simulink model "my_buck_nn_5_10"  (R2021a)
settings: Solver=ode8  StartTime=0.0  StopTime=T  RelTol=1e-3  EnableMultiTasking=on
undefined symbols (not defined in the file): a00c, a00o, a01c, a01o, a10c, a10o, a11c, a11o, b0c, b0o, b1c, b1o, i0, T_sw, v0
libraries: neural x57, simulink x1
(part 2 of 2)

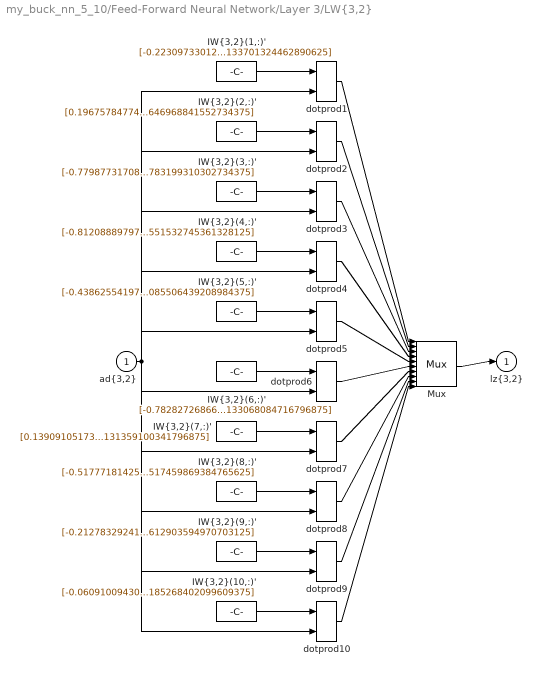
== system my_buck_nn_5_10/Feed-Forward Neural Network/Layer 3/LW{3,2} ==
  "ad{3,2}" : Inport  PortDimensions=10
      mask Display: e = 0.06;c1 = [120 230 180]/255;c2 = ([120 230 180]+0)/(256+128);c3 = ([120 230 180]+128)/(256+128);patch([0 1 1 0],[0 0 1 1],c1);patch([0 1 1 1-e 1-e 0+e],[0 0 1 1-e 0+e 0+e],c2);patch([0 0 1 1-e 0+e 0+e],[0 1 1 1-e 1-e 0+e],c3);plot([0 1 1 0 0],[0 0 1 1 0]);
  "IW{3,2}(1,:)'" : Constant  Value=[-0.2230973301246004236730868797167204320430755615234375;-0.7932748282150023921843740026815794408321380615234375;0.79085097892476452496879346654168330132961273193359375;-0.70189923383787033994707371675758622586727142333984375;-0.989793512776859785162741900421679019927978515625;-0.25570181827175486599657006081542931497097015380859375;-0.4845417555697097977684961733757518231868743896484375;-0.03901169535660164999768539928481914103031158447265625;-0.1497645933363858095077603138634003698825836181640625;0.5126260157213560209044089788221754133701324462890625]
      mask Display: e = 0.06;c1 = [120 150 230]/255;c2 = ([120 150 230]+0)/383;c3 = ([120 150 230]+128)/383;patch([0 1 1 0],[0 0 1 1],c1);patch([0 1 1 1-e 1-e 0+e],[0 0 1 1-e 0+e 0+e],c2);patch([0 0 1 1-e 0+e 0+e],[0 1 1 1-e 1-e 0+e],c3);plot([0 1 1 0 0],[0 0 1 1 0]);disp('weights');
  "IW{3,2}(10,:)'" : Constant  Value=[-0.0609100943023948016019630813389085233211517333984375;-0.80372367245294196180793733219616115093231201171875;0.27081599181474358406518376796157099306583404541015625;0.265189392929031431123121365089900791645050048828125;-0.7240301944141958045975115965120494365692138671875;-0.57188810753222940608253566097118891775608062744140625;0.55258359868805495551669082487933337688446044921875;-0.40945653303743967388328428569366224110126495361328125;-0.7914296649209917600131802828400395810604095458984375;-0.33082945599161239780272580901510082185268402099609375]
      mask Display: e = 0.06;c1 = [120 150 230]/255;c2 = ([120 150 230]+0)/383;c3 = ([120 150 230]+128)/383;patch([0 1 1 0],[0 0 1 1],c1);patch([0 1 1 1-e 1-e 0+e],[0 0 1 1-e 0+e 0+e],c2);patch([0 0 1 1-e 0+e 0+e],[0 1 1 1-e 1-e 0+e],c3);plot([0 1 1 0 0],[0 0 1 1 0]);disp('weights');
  "IW{3,2}(2,:)'" : Constant  Value=[0.196757847742274893931835322291590273380279541015625;0.6454480727285536456605541388853453099727630615234375;0.99750915171941356707208115039975382387638092041015625;0.827041936661400800545607125968672335147857666015625;0.0417420581953746872017063651583157479763031005859375;1.0293967746717260780542346765287220478057861328125;0.00641324259274966834709630347788333892822265625;-0.09573473684369075697997431007024715654551982879638671875;-0.2787173553106720991223710370832122862339019775390625;-0.260939600114958147880628303028061054646968841552734375]
      mask Display: e = 0.06;c1 = [120 150 230]/255;c2 = ([120 150 230]+0)/383;c3 = ([120 150 230]+128)/383;patch([0 1 1 0],[0 0 1 1],c1);patch([0 1 1 1-e 1-e 0+e],[0 0 1 1-e 0+e 0+e],c2);patch([0 0 1 1-e 0+e 0+e],[0 1 1 1-e 1-e 0+e],c3);plot([0 1 1 0 0],[0 0 1 1 0]);disp('weights');
  "IW{3,2}(3,:)'" : Constant  Value=[-0.779877317085582166811263959971256554126739501953125;-0.310071870090603274316976012414670549333095550537109375;0.72432386795238923316020418496918864548206329345703125;0.419290922552696176950348672107793390750885009765625;-0.56736289194307421013263592612929642200469970703125;-0.3526319020860426700636480745743028819561004638671875;0.3565431330236761287011404419899918138980865478515625;1.246137269856822715752286967472173273563385009765625;-0.8664588759141953477893594026681967079639434814453125;0.1539704729454270670796489639542414806783199310302734375]
      mask Display: e = 0.06;c1 = [120 150 230]/255;c2 = ([120 150 230]+0)/383;c3 = ([120 150 230]+128)/383;patch([0 1 1 0],[0 0 1 1],c1);patch([0 1 1 1-e 1-e 0+e],[0 0 1 1-e 0+e 0+e],c2);patch([0 0 1 1-e 0+e 0+e],[0 1 1 1-e 1-e 0+e],c3);plot([0 1 1 0 0],[0 0 1 1 0]);disp('weights');
  "IW{3,2}(4,:)'" : Constant  Value=[-0.8120888979725917611318664057762362062931060791015625;0.6989923138619509312974287240649573504924774169921875;-0.8092821167810611004966858672560192644596099853515625;0.9321006564887095446891862593474797904491424560546875;-0.47196353282645731042066472582519054412841796875;-0.7802084968839901879533726969384588301181793212890625;0.5970384044771872567025639000348746776580810546875;0.695697603264001873668576081399805843830108642578125;-0.657985029570661961173527743085287511348724365234375;-0.92353117770848058842858563366462476551532745361328125]
      mask Display: e = 0.06;c1 = [120 150 230]/255;c2 = ([120 150 230]+0)/383;c3 = ([120 150 230]+128)/383;patch([0 1 1 0],[0 0 1 1],c1);patch([0 1 1 1-e 1-e 0+e],[0 0 1 1-e 0+e 0+e],c2);patch([0 0 1 1-e 0+e 0+e],[0 1 1 1-e 1-e 0+e],c3);plot([0 1 1 0 0],[0 0 1 1 0]);disp('weights');
  "IW{3,2}(5,:)'" : Constant  Value=[-0.438625541976773281049872821313329041004180908203125;-0.83434166362172679232145355854299850761890411376953125;-0.10138351170699401448960230709417373873293399810791015625;-0.7312618806762001266719153136364184319972991943359375;-0.290691564768943866425843225442804396152496337890625;-0.03730485749667165895626652627470321021974086761474609375;0.502479013885176239995189462206326425075531005859375;0.445592640810527129691109848863561637699604034423828125;0.53963122023129361792825875454582273960113525390625;-0.75669893589882464279838814036338590085506439208984375]
      mask Display: e = 0.06;c1 = [120 150 230]/255;c2 = ([120 150 230]+0)/383;c3 = ([120 150 230]+128)/383;patch([0 1 1 0],[0 0 1 1],c1);patch([0 1 1 1-e 1-e 0+e],[0 0 1 1-e 0+e 0+e],c2);patch([0 0 1 1-e 0+e 0+e],[0 1 1 1-e 1-e 0+e],c3);plot([0 1 1 0 0],[0 0 1 1 0]);disp('weights');
  "IW{3,2}(6,:)'" : Constant  Value=[-0.7828272686657609114035949460230767726898193359375;-0.8950889462309967736786120440228842198848724365234375;0.96021626961651695975064058075076900422573089599609375;-0.4361700008671605122145820132573135197162628173828125;-0.72811329607470209879238609573803842067718505859375;0.78059976706595379791764344190596602857112884521484375;-0.0663312268493079226772124457056634128093719482421875;-0.4842613379382820770757689388119615614414215087890625;0.914253204482205372727321446291171014308929443359375;-0.90156556177200986024189433010178618133068084716796875]
      mask Display: e = 0.06;c1 = [120 150 230]/255;c2 = ([120 150 230]+0)/383;c3 = ([120 150 230]+128)/383;patch([0 1 1 0],[0 0 1 1],c1);patch([0 1 1 1-e 1-e 0+e],[0 0 1 1-e 0+e 0+e],c2);patch([0 0 1 1-e 0+e 0+e],[0 1 1 1-e 1-e 0+e],c3);plot([0 1 1 0 0],[0 0 1 1 0]);disp('weights');
  "IW{3,2}(7,:)'" : Constant  Value=[0.13909105173843716585224683512933552265167236328125;0.75522199756791630331775877493782900273799896240234375;0.9269594132792653429220308680669404566287994384765625;-0.925064417004890504614422752638347446918487548828125;0.9889470498369294926277461854624561965465545654296875;0.99295289620838256272605804042541421949863433837890625;-0.381661240820658775874107959680259227752685546875;-0.50378735118134054804528432214283384382724761962890625;0.471059893245600047606558291590772569179534912109375;-0.73205460720426163145901909956592135131359100341796875]
      mask Display: e = 0.06;c1 = [120 150 230]/255;c2 = ([120 150 230]+0)/383;c3 = ([120 150 230]+128)/383;patch([0 1 1 0],[0 0 1 1],c1);patch([0 1 1 1-e 1-e 0+e],[0 0 1 1-e 0+e 0+e],c2);patch([0 0 1 1-e 0+e 0+e],[0 1 1 1-e 1-e 0+e],c3);plot([0 1 1 0 0],[0 0 1 1 0]);disp('weights');
  "IW{3,2}(8,:)'" : Constant  Value=[-0.5177718142514573518297993359738029539585113525390625;0.58233364417824284853253402616246603429317474365234375;-0.82418594893296648340452748016105033457279205322265625;-0.1877319934952508539982574120585923083126544952392578125;-0.1058780985460454626689852375420741736888885498046875;-0.450030200081221576358103675374877639114856719970703125;0.2461491554452306385059046078822575509548187255859375;0.8445581490884281894437890514382161200046539306640625;-0.06654864536490290305437156348489224910736083984375;0.5417979307102049890687567312852479517459869384765625]
      mask Display: e = 0.06;c1 = [120 150 230]/255;c2 = ([120 150 230]+0)/383;c3 = ([120 150 230]+128)/383;patch([0 1 1 0],[0 0 1 1],c1);patch([0 1 1 1-e 1-e 0+e],[0 0 1 1-e 0+e 0+e],c2);patch([0 0 1 1-e 0+e 0+e],[0 1 1 1-e 1-e 0+e],c3);plot([0 1 1 0 0],[0 0 1 1 0]);disp('weights');
  "IW{3,2}(9,:)'" : Constant  Value=[-0.2127832924122099456099022063426673412322998046875;0.0299459590999605375361003467560294666327536106109619140625;-0.351824095765843558591967621396179310977458953857421875;-0.9245459727240372682643965163151733577251434326171875;0.62369822352246284680177268455736339092254638671875;0.90248600905930087545669948667637072503566741943359375;-0.5037594788739097051433191154501400887966156005859375;0.385035381831421774645463074193685315549373626708984375;-0.4523169523443575368304436778998933732509613037109375;0.333631398082735952659305667111766524612903594970703125]
      mask Display: e = 0.06;c1 = [120 150 230]/255;c2 = ([120 150 230]+0)/383;c3 = ([120 150 230]+128)/383;patch([0 1 1 0],[0 0 1 1],c1);patch([0 1 1 1-e 1-e 0+e],[0 0 1 1-e 0+e 0+e],c2);patch([0 0 1 1-e 0+e 0+e],[0 1 1 1-e 1-e 0+e],c3);plot([0 1 1 0 0],[0 0 1 1 0]);disp('weights');
  Mux : Mux  Inputs=10
      mask Display: e = 0.06;c1 = [120 150 230]/255;c2 = ([120 150 230]+0)/383;c3 = ([120 150 230]+128)/383;patch([0 1 1 0],[0 0 1 1],c1);patch([0 1 1 1-e 1-e 0+e],[0 0 1 1-e 0+e 0+e],c2);patch([0 0 1 1-e 0+e 0+e],[0 1 1 1-e 1-e 0+e],c3);plot([0 1 1 0 0],[0 0 1 1 0]);disp('Mux');
  dotprod{1..10} (10 alike) : neural/Weight Functions/dotprod
  "lz{3,2}" : Outport
      mask Display: e = 0.06;c1 = [120 230 180]/255;c2 = ([120 230 180]+0)/(256+128);c3 = ([120 230 180]+128)/(256+128);patch([0 1 1 0],[0 0 1 1],c1);patch([0 1 1 1-e 1-e 0+e],[0 0 1 1-e 0+e 0+e],c2);patch([0 0 1 1-e 0+e 0+e],[0 1 1 1-e 1-e 0+e],c3);plot([0 1 1 0 0],[0 0 1 1 0]);
  wires:
  "IW{3,2}(1,:)'"/1 -> dotprod1/1
  "ad{3,2}"/1 -> dotprod1/2, dotprod2/2, dotprod3/2, dotprod4/2, dotprod5/2, dotprod6/2, dotprod7/2, dotprod8/2, dotprod9/2, dotprod10/2
  dotprod1/1 -> Mux/1
  "IW{3,2}(2,:)'"/1 -> dotprod2/1
  dotprod2/1 -> Mux/2
  "IW{3,2}(3,:)'"/1 -> dotprod3/1
  dotprod3/1 -> Mux/3
  "IW{3,2}(4,:)'"/1 -> dotprod4/1
  dotprod4/1 -> Mux/4
  "IW{3,2}(5,:)'"/1 -> dotprod5/1
  dotprod5/1 -> Mux/5
  "IW{3,2}(6,:)'"/1 -> dotprod6/1
  dotprod6/1 -> Mux/6
  "IW{3,2}(7,:)'"/1 -> dotprod7/1
  dotprod7/1 -> Mux/7
  "IW{3,2}(8,:)'"/1 -> dotprod8/1
  dotprod8/1 -> Mux/8
  "IW{3,2}(9,:)'"/1 -> dotprod9/1
  dotprod9/1 -> Mux/9
  "IW{3,2}(10,:)'"/1 -> dotprod10/1
  dotprod10/1 -> Mux/10
  Mux/1 -> "lz{3,2}"/1

== system my_buck_nn_5_10/Feed-Forward Neural Network/Layer 4/Delays 1 ==
  "p{4}" : Inport  PortDimensions=10
      mask Display: e = 0.06;c1 = [120 230 180]/255;c2 = ([120 230 180]+0)/(256+128);c3 = ([120 230 180]+128)/(256+128);patch([0 1 1 0],[0 0 1 1],c1);patch([0 1 1 1-e 1-e 0+e],[0 0 1 1-e 0+e 0+e],c2);patch([0 0 1 1-e 0+e 0+e],[0 1 1 1-e 1-e 0+e],c3);plot([0 1 1 0 0],[0 0 1 1 0]);
  mux : Mux  Inputs=1
      mask Display: e = 0.06;c1 = [120 150 230]/255;c2 = ([120 150 230]+0)/383;c3 = ([120 150 230]+128)/383;patch([0 1 1 0],[0 0 1 1],c1);patch([0 1 1 1-e 1-e 0+e],[0 0 1 1-e 0+e 0+e],c2);patch([0 0 1 1-e 0+e 0+e],[0 1 1 1-e 1-e 0+e],c3);plot([0 1 1 0 0],[0 0 1 1 0]);disp('Mux')
  "pd{4,3}" : Outport
      mask Display: e = 0.06;c1 = [120 230 180]/255;c2 = ([120 230 180]+0)/(256+128);c3 = ([120 230 180]+128)/(256+128);patch([0 1 1 0],[0 0 1 1],c1);patch([0 1 1 1-e 1-e 0+e],[0 0 1 1-e 0+e 0+e],c2);patch([0 0 1 1-e 0+e 0+e],[0 1 1 1-e 1-e 0+e],c3);plot([0 1 1 0 0],[0 0 1 1 0]);
  wires:
  "p{4}"/1 -> mux/1
  mux/1 -> "pd{4,3}"/1

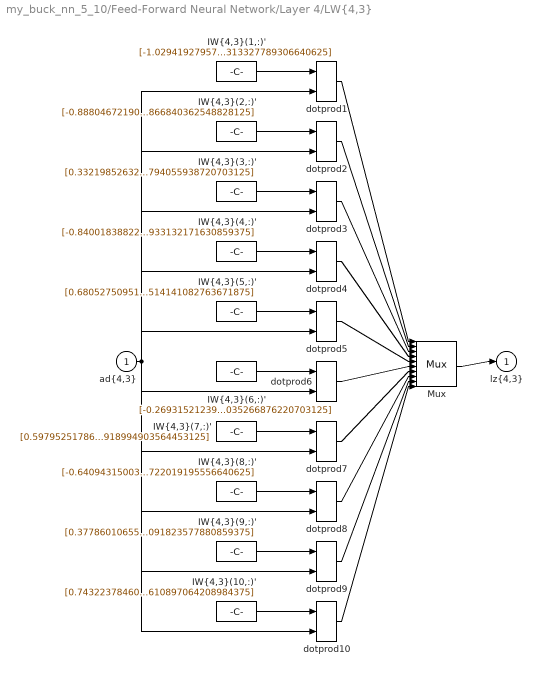
== system my_buck_nn_5_10/Feed-Forward Neural Network/Layer 4/LW{4,3} ==
  "ad{4,3}" : Inport  PortDimensions=10
      mask Display: e = 0.06;c1 = [120 230 180]/255;c2 = ([120 230 180]+0)/(256+128);c3 = ([120 230 180]+128)/(256+128);patch([0 1 1 0],[0 0 1 1],c1);patch([0 1 1 1-e 1-e 0+e],[0 0 1 1-e 0+e 0+e],c2);patch([0 0 1 1-e 0+e 0+e],[0 1 1 1-e 1-e 0+e],c3);plot([0 1 1 0 0],[0 0 1 1 0]);
  "IW{4,3}(1,:)'" : Constant  Value=[-1.0294192795749570468188949234900064766407012939453125;-0.90361251400663800126267233281396329402923583984375;0.4150520984028307491797704642522148787975311279296875;1.116263420383598603535801885300315916538238525390625;0.51535515438125945042457942690816707909107208251953125;-0.27657443793255886976822921496932394802570343017578125;0.8017198878994455935043106364901177585124969482421875;0.90736871796228657505167802810319699347019195556640625;0.8583396849382116666760111911571584641933441162109375;0.4555384430431816955575641259201802313327789306640625]
      mask Display: e = 0.06;c1 = [120 150 230]/255;c2 = ([120 150 230]+0)/383;c3 = ([120 150 230]+128)/383;patch([0 1 1 0],[0 0 1 1],c1);patch([0 1 1 1-e 1-e 0+e],[0 0 1 1-e 0+e 0+e],c2);patch([0 0 1 1-e 0+e 0+e],[0 1 1 1-e 1-e 0+e],c3);plot([0 1 1 0 0],[0 0 1 1 0]);disp('weights');
  "IW{4,3}(10,:)'" : Constant  Value=[0.7432237846080251841840436100028455257415771484375;0.46893960209625651369691468062228523194789886474609375;-0.0028141976625353291689701773492515712860040366649627685546875;0.00826864527001815174944709951887489296495914459228515625;-0.84677144199838150218084820153308100998401641845703125;0.485639008338516975360477090362110175192356109619140625;0.75219548697486426913627610701951198279857635498046875;-0.07004352274760765328931455542260664515197277069091796875;-0.7970138027155677651336418421124108135700225830078125;-0.69103412382015871884277657954953610897064208984375]
      mask Display: e = 0.06;c1 = [120 150 230]/255;c2 = ([120 150 230]+0)/383;c3 = ([120 150 230]+128)/383;patch([0 1 1 0],[0 0 1 1],c1);patch([0 1 1 1-e 1-e 0+e],[0 0 1 1-e 0+e 0+e],c2);patch([0 0 1 1-e 0+e 0+e],[0 1 1 1-e 1-e 0+e],c3);plot([0 1 1 0 0],[0 0 1 1 0]);disp('weights');
  "IW{4,3}(2,:)'" : Constant  Value=[-0.888046721906101677035394459380768239498138427734375;0.0726379653884623721626923043004353530704975128173828125;0.9453236936730438078058114115265198051929473876953125;0.2494443433817846444977561759515083394944667816162109375;0.220809445203211052177749706970644183456897735595703125;0.289920687041711755416173446064931340515613555908203125;0.5613608682756072720820839094812981784343719482421875;0.341075314816695396302748122252523899078369140625;0.49429319948021177566488404409028589725494384765625;-0.71248931176412455545943203105707652866840362548828125]
      mask Display: e = 0.06;c1 = [120 150 230]/255;c2 = ([120 150 230]+0)/383;c3 = ([120 150 230]+128)/383;patch([0 1 1 0],[0 0 1 1],c1);patch([0 1 1 1-e 1-e 0+e],[0 0 1 1-e 0+e 0+e],c2);patch([0 0 1 1-e 0+e 0+e],[0 1 1 1-e 1-e 0+e],c3);plot([0 1 1 0 0],[0 0 1 1 0]);disp('weights');
  "IW{4,3}(3,:)'" : Constant  Value=[0.332198526327468213192872781291953288018703460693359375;-0.75808586022752721955697552402853034436702728271484375;0.7905101121742210690257479654974304139614105224609375;0.9515285630258107918422183502116240561008453369140625;0.4532613166552452721447252770303748548030853271484375;0.1603085629507346177025084443812374956905841827392578125;0.3964781030208801571035337474313564598560333251953125;-0.5420869984389022899762267115875147283077239990234375;-0.267533503745900180792460787415620870888233184814453125;-0.0578756029610672240170998747998964972794055938720703125]
      mask Display: e = 0.06;c1 = [120 150 230]/255;c2 = ([120 150 230]+0)/383;c3 = ([120 150 230]+128)/383;patch([0 1 1 0],[0 0 1 1],c1);patch([0 1 1 1-e 1-e 0+e],[0 0 1 1-e 0+e 0+e],c2);patch([0 0 1 1-e 0+e 0+e],[0 1 1 1-e 1-e 0+e],c3);plot([0 1 1 0 0],[0 0 1 1 0]);disp('weights');
  "IW{4,3}(4,:)'" : Constant  Value=[-0.8400183882260403578356999787501990795135498046875;-0.9003158720653912094888937645009718835353851318359375;0.0447282758989089312962050826172344386577606201171875;-0.5500400201876016748059328165254555642604827880859375;-0.22505454418855297404888915480114519596099853515625;0.1298653965160305734372059305314905941486358642578125;-0.579414417456753039203931621159426867961883544921875;-0.1909900735982164032833452438353560864925384521484375;-0.5286799665021693073185815592296421527862548828125;-0.1828468925020911850509719442925415933132171630859375]
      mask Display: e = 0.06;c1 = [120 150 230]/255;c2 = ([120 150 230]+0)/383;c3 = ([120 150 230]+128)/383;patch([0 1 1 0],[0 0 1 1],c1);patch([0 1 1 1-e 1-e 0+e],[0 0 1 1-e 0+e 0+e],c2);patch([0 0 1 1-e 0+e 0+e],[0 1 1 1-e 1-e 0+e],c3);plot([0 1 1 0 0],[0 0 1 1 0]);disp('weights');
  "IW{4,3}(5,:)'" : Constant  Value=[0.68052750951113283317539526251493953168392181396484375;0.38999493535865925597505565747269429266452789306640625;0.89194180381809851088092955251340754330158233642578125;-0.84634114970135387867600229583331383764743804931640625;0.80110951928757001549996630274108611047267913818359375;-0.95060536619847957329199061859981156885623931884765625;-0.98551110499143879106753729502088390290737152099609375;0.027213592663299944474086800028089783154428005218505859375;-0.187096629681309967185853793125716038048267364501953125;-0.84249727126052220693708250109921209514141082763671875]
      mask Display: e = 0.06;c1 = [120 150 230]/255;c2 = ([120 150 230]+0)/383;c3 = ([120 150 230]+128)/383;patch([0 1 1 0],[0 0 1 1],c1);patch([0 1 1 1-e 1-e 0+e],[0 0 1 1-e 0+e 0+e],c2);patch([0 0 1 1-e 0+e 0+e],[0 1 1 1-e 1-e 0+e],c3);plot([0 1 1 0 0],[0 0 1 1 0]);disp('weights');
  "IW{4,3}(6,:)'" : Constant  Value=[-0.26931521239965461322896089768619276583194732666015625;0.427806189782669099574974325150833465158939361572265625;0.48318366738745555100109640989103354513645172119140625;0.28362423213139742461663672656868584454059600830078125;-0.32126802511794905203856842490495182573795318603515625;0.436368053411835654653572191818966530263423919677734375;0.53198208490043674689928820953355170786380767822265625;0.497747808237356093030712145264260470867156982421875;0.79303149481026558031970807860489003360271453857421875;0.370495148788917927351604930663597770035266876220703125]
      mask Display: e = 0.06;c1 = [120 150 230]/255;c2 = ([120 150 230]+0)/383;c3 = ([120 150 230]+128)/383;patch([0 1 1 0],[0 0 1 1],c1);patch([0 1 1 1-e 1-e 0+e],[0 0 1 1-e 0+e 0+e],c2);patch([0 0 1 1-e 0+e 0+e],[0 1 1 1-e 1-e 0+e],c3);plot([0 1 1 0 0],[0 0 1 1 0]);disp('weights');
  "IW{4,3}(7,:)'" : Constant  Value=[0.5979525178645783700659421810996718704700469970703125;-0.14159483129974059778533046483062207698822021484375;-0.6776594763368908314049576802062802016735076904296875;0.50262767158160936986632805201224982738494873046875;-0.846414497423427558686626070993952453136444091796875;-0.0643648894747215205569546014885418117046356201171875;-0.589090060829402517583730514161288738250732421875;-0.1568336303035640089120761331287212669849395751953125;-0.8195438534386401130404919967986643314361572265625;-0.832104792336839427235872790333814918994903564453125]
      mask Display: e = 0.06;c1 = [120 150 230]/255;c2 = ([120 150 230]+0)/383;c3 = ([120 150 230]+128)/383;patch([0 1 1 0],[0 0 1 1],c1);patch([0 1 1 1-e 1-e 0+e],[0 0 1 1-e 0+e 0+e],c2);patch([0 0 1 1-e 0+e 0+e],[0 1 1 1-e 1-e 0+e],c3);plot([0 1 1 0 0],[0 0 1 1 0]);disp('weights');
  "IW{4,3}(8,:)'" : Constant  Value=[-0.6409431500377513746258273386047221720218658447265625;0.1883066998060323182784259188338182866573333740234375;-0.916856114885365780509118849295191466808319091796875;0.12853055012930614253718886175192892551422119140625;-0.7133452264178103963132571152527816593647003173828125;0.95196949779569184357796984841115772724151611328125;-0.7552758183154846260976000849041156470775604248046875;0.1186967978556603409145964178605936467647552490234375;-0.8085605744758110891012847787351347506046295166015625;0.377040554206902189804395675309933722019195556640625]
      mask Display: e = 0.06;c1 = [120 150 230]/255;c2 = ([120 150 230]+0)/383;c3 = ([120 150 230]+128)/383;patch([0 1 1 0],[0 0 1 1],c1);patch([0 1 1 1-e 1-e 0+e],[0 0 1 1-e 0+e 0+e],c2);patch([0 0 1 1-e 0+e 0+e],[0 1 1 1-e 1-e 0+e],c3);plot([0 1 1 0 0],[0 0 1 1 0]);disp('weights');
  "IW{4,3}(9,:)'" : Constant  Value=[0.3778601065503313094495752011425793170928955078125;-0.029141535279670005564867096836678683757781982421875;-0.9357879927942480691172022488899528980255126953125;0.7570712668526395905388426399440504610538482666015625;0.139407147217721405496604347717948257923126220703125;-0.82210386114964695281059903209097683429718017578125;0.64836927764665031048707533045671880245208740234375;-0.271775265713698477298976285965181887149810791015625;0.5324504787258648175196640295325778424739837646484375;-0.070113573866945611001710858545266091823577880859375]
      mask Display: e = 0.06;c1 = [120 150 230]/255;c2 = ([120 150 230]+0)/383;c3 = ([120 150 230]+128)/383;patch([0 1 1 0],[0 0 1 1],c1);patch([0 1 1 1-e 1-e 0+e],[0 0 1 1-e 0+e 0+e],c2);patch([0 0 1 1-e 0+e 0+e],[0 1 1 1-e 1-e 0+e],c3);plot([0 1 1 0 0],[0 0 1 1 0]);disp('weights');
  Mux : Mux  Inputs=10
      mask Display: e = 0.06;c1 = [120 150 230]/255;c2 = ([120 150 230]+0)/383;c3 = ([120 150 230]+128)/383;patch([0 1 1 0],[0 0 1 1],c1);patch([0 1 1 1-e 1-e 0+e],[0 0 1 1-e 0+e 0+e],c2);patch([0 0 1 1-e 0+e 0+e],[0 1 1 1-e 1-e 0+e],c3);plot([0 1 1 0 0],[0 0 1 1 0]);disp('Mux');
  dotprod{1..10} (10 alike) : neural/Weight Functions/dotprod
  "lz{4,3}" : Outport
      mask Display: e = 0.06;c1 = [120 230 180]/255;c2 = ([120 230 180]+0)/(256+128);c3 = ([120 230 180]+128)/(256+128);patch([0 1 1 0],[0 0 1 1],c1);patch([0 1 1 1-e 1-e 0+e],[0 0 1 1-e 0+e 0+e],c2);patch([0 0 1 1-e 0+e 0+e],[0 1 1 1-e 1-e 0+e],c3);plot([0 1 1 0 0],[0 0 1 1 0]);
  wires:
  "IW{4,3}(1,:)'"/1 -> dotprod1/1
  "ad{4,3}"/1 -> dotprod1/2, dotprod2/2, dotprod3/2, dotprod4/2, dotprod5/2, dotprod6/2, dotprod7/2, dotprod8/2, dotprod9/2, dotprod10/2
  dotprod1/1 -> Mux/1
  "IW{4,3}(2,:)'"/1 -> dotprod2/1
  dotprod2/1 -> Mux/2
  "IW{4,3}(3,:)'"/1 -> dotprod3/1
  dotprod3/1 -> Mux/3
  "IW{4,3}(4,:)'"/1 -> dotprod4/1
  dotprod4/1 -> Mux/4
  "IW{4,3}(5,:)'"/1 -> dotprod5/1
  dotprod5/1 -> Mux/5
  "IW{4,3}(6,:)'"/1 -> dotprod6/1
  dotprod6/1 -> Mux/6
  "IW{4,3}(7,:)'"/1 -> dotprod7/1
  dotprod7/1 -> Mux/7
  "IW{4,3}(8,:)'"/1 -> dotprod8/1
  dotprod8/1 -> Mux/8
  "IW{4,3}(9,:)'"/1 -> dotprod9/1
  dotprod9/1 -> Mux/9
  "IW{4,3}(10,:)'"/1 -> dotprod10/1
  dotprod10/1 -> Mux/10
  Mux/1 -> "lz{4,3}"/1

== system my_buck_nn_5_10/Feed-Forward Neural Network/Layer 5/Delays 1 ==
  "p{5}" : Inport  PortDimensions=10
      mask Display: e = 0.06;c1 = [120 230 180]/255;c2 = ([120 230 180]+0)/(256+128);c3 = ([120 230 180]+128)/(256+128);patch([0 1 1 0],[0 0 1 1],c1);patch([0 1 1 1-e 1-e 0+e],[0 0 1 1-e 0+e 0+e],c2);patch([0 0 1 1-e 0+e 0+e],[0 1 1 1-e 1-e 0+e],c3);plot([0 1 1 0 0],[0 0 1 1 0]);
  mux : Mux  Inputs=1
      mask Display: e = 0.06;c1 = [120 150 230]/255;c2 = ([120 150 230]+0)/383;c3 = ([120 150 230]+128)/383;patch([0 1 1 0],[0 0 1 1],c1);patch([0 1 1 1-e 1-e 0+e],[0 0 1 1-e 0+e 0+e],c2);patch([0 0 1 1-e 0+e 0+e],[0 1 1 1-e 1-e 0+e],c3);plot([0 1 1 0 0],[0 0 1 1 0]);disp('Mux')
  "pd{5,4}" : Outport
      mask Display: e = 0.06;c1 = [120 230 180]/255;c2 = ([120 230 180]+0)/(256+128);c3 = ([120 230 180]+128)/(256+128);patch([0 1 1 0],[0 0 1 1],c1);patch([0 1 1 1-e 1-e 0+e],[0 0 1 1-e 0+e 0+e],c2);patch([0 0 1 1-e 0+e 0+e],[0 1 1 1-e 1-e 0+e],c3);plot([0 1 1 0 0],[0 0 1 1 0]);
  wires:
  "p{5}"/1 -> mux/1
  mux/1 -> "pd{5,4}"/1

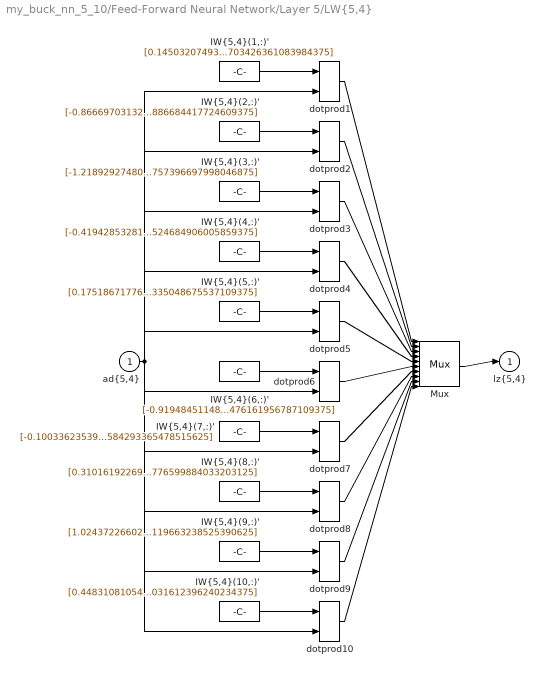
== system my_buck_nn_5_10/Feed-Forward Neural Network/Layer 5/LW{5,4} ==
  "ad{5,4}" : Inport  PortDimensions=10
      mask Display: e = 0.06;c1 = [120 230 180]/255;c2 = ([120 230 180]+0)/(256+128);c3 = ([120 230 180]+128)/(256+128);patch([0 1 1 0],[0 0 1 1],c1);patch([0 1 1 1-e 1-e 0+e],[0 0 1 1-e 0+e 0+e],c2);patch([0 0 1 1-e 0+e 0+e],[0 1 1 1-e 1-e 0+e],c3);plot([0 1 1 0 0],[0 0 1 1 0]);
  "IW{5,4}(1,:)'" : Constant  Value=[0.1450320749354816751708341371340793557465076446533203125;0.0627214805959988297434648529815603978931903839111328125;0.298067758339173705106617262572399340569972991943359375;-0.0548090595133305935604539627092890441417694091796875;0.497579072825059309792550266138277947902679443359375;0.58497699526499935540613250850583426654338836669921875;-0.7981215550258102808811599970795214176177978515625;0.16355693303256657600286416709423065185546875;0.442469893838695060850341178593225777149200439453125;-0.8790057296612390214107790598063729703426361083984375]
      mask Display: e = 0.06;c1 = [120 150 230]/255;c2 = ([120 150 230]+0)/383;c3 = ([120 150 230]+128)/383;patch([0 1 1 0],[0 0 1 1],c1);patch([0 1 1 1-e 1-e 0+e],[0 0 1 1-e 0+e 0+e],c2);patch([0 0 1 1-e 0+e 0+e],[0 1 1 1-e 1-e 0+e],c3);plot([0 1 1 0 0],[0 0 1 1 0]);disp('weights');
  "IW{5,4}(10,:)'" : Constant  Value=[0.4483108105498885276318787873606197535991668701171875;-0.99330323242137108508131859707646071910858154296875;-0.246240956167785185471075237728655338287353515625;-0.3874554233376514833508963420172221958637237548828125;0.2242160508367010418595555165666155517101287841796875;-0.4848762167316504889669204203528352081775665283203125;-0.3317733347594324921914221704355441033840179443359375;-0.7043715041006286536884317683870904147624969482421875;0.7389134246882402834444292238913476467132568359375;-0.635961534589293275843147057457827031612396240234375]
      mask Display: e = 0.06;c1 = [120 150 230]/255;c2 = ([120 150 230]+0)/383;c3 = ([120 150 230]+128)/383;patch([0 1 1 0],[0 0 1 1],c1);patch([0 1 1 1-e 1-e 0+e],[0 0 1 1-e 0+e 0+e],c2);patch([0 0 1 1-e 0+e 0+e],[0 1 1 1-e 1-e 0+e],c3);plot([0 1 1 0 0],[0 0 1 1 0]);disp('weights');
  "IW{5,4}(2,:)'" : Constant  Value=[-0.86669703132327857719729991003987379372119903564453125;0.269149987761666376062663630364113487303256988525390625;-0.8808628596725751602747322976938448846340179443359375;-0.3838244718805541300099548607249744236469268798828125;-0.91457026360075455162501611994230188429355621337890625;0.973736353898714046550821876735426485538482666015625;-0.6482863157603888648594647747813723981380462646484375;-0.649600911117570678499077985179610550403594970703125;0.865086618454026012869917394709773361682891845703125;0.64501588533845843898006933159194886684417724609375]
      mask Display: e = 0.06;c1 = [120 150 230]/255;c2 = ([120 150 230]+0)/383;c3 = ([120 150 230]+128)/383;patch([0 1 1 0],[0 0 1 1],c1);patch([0 1 1 1-e 1-e 0+e],[0 0 1 1-e 0+e 0+e],c2);patch([0 0 1 1-e 0+e 0+e],[0 1 1 1-e 1-e 0+e],c3);plot([0 1 1 0 0],[0 0 1 1 0]);disp('weights');
  "IW{5,4}(3,:)'" : Constant  Value=[-1.21892927480441048970760675729252398014068603515625;0.383625134676446932768811848291079513728618621826171875;0.327319401269074827798277738111210055649280548095703125;-0.19158734413444111766011701547540724277496337890625;0.55104250605665516804521075755474157631397247314453125;0.80821710490659859349449334331438876688480377197265625;0.2001682445535613030784816146478988230228424072265625;0.0345780393415269227119779316126368939876556396484375;0.91020064001060774216966819949448108673095703125;-0.3280584950662184251513053823146037757396697998046875]
      mask Display: e = 0.06;c1 = [120 150 230]/255;c2 = ([120 150 230]+0)/383;c3 = ([120 150 230]+128)/383;patch([0 1 1 0],[0 0 1 1],c1);patch([0 1 1 1-e 1-e 0+e],[0 0 1 1-e 0+e 0+e],c2);patch([0 0 1 1-e 0+e 0+e],[0 1 1 1-e 1-e 0+e],c3);plot([0 1 1 0 0],[0 0 1 1 0]);disp('weights');
  "IW{5,4}(4,:)'" : Constant  Value=[-0.4194285328103266596855291936662979423999786376953125;-0.4522345211725362634780367443454451858997344970703125;0.426790225335050621424670680426061153411865234375;-0.1111418378957067520929058446199633181095123291015625;-0.244396270181673980204095641965977847576141357421875;0.0793646474432037063451161884586326777935028076171875;-0.8314968589339566396034797435277141630649566650390625;0.60270078275166039105670279241167008876800537109375;0.13359844665376652272925639408640563488006591796875;-0.29055164649179854308158610365353524684906005859375]
      mask Display: e = 0.06;c1 = [120 150 230]/255;c2 = ([120 150 230]+0)/383;c3 = ([120 150 230]+128)/383;patch([0 1 1 0],[0 0 1 1],c1);patch([0 1 1 1-e 1-e 0+e],[0 0 1 1-e 0+e 0+e],c2);patch([0 0 1 1-e 0+e 0+e],[0 1 1 1-e 1-e 0+e],c3);plot([0 1 1 0 0],[0 0 1 1 0]);disp('weights');
  "IW{5,4}(5,:)'" : Constant  Value=[0.1751867177654597984570727930986322462558746337890625;-0.3296854842657210848955173787544481456279754638671875;-0.2241343517844553989704081686795689165592193603515625;0.124900000865647786696399634820409119129180908203125;0.4159022013891300328936040386906825006008148193359375;-0.46003582159032152532063264516182243824005126953125;0.8727309990640035319842127137235365808010101318359375;-0.5035489178254646258636739730718545615673065185546875;-0.9181575828472128275592467616661451756954193115234375;-0.658748669323235613859424120164476335048675537109375]
      mask Display: e = 0.06;c1 = [120 150 230]/255;c2 = ([120 150 230]+0)/383;c3 = ([120 150 230]+128)/383;patch([0 1 1 0],[0 0 1 1],c1);patch([0 1 1 1-e 1-e 0+e],[0 0 1 1-e 0+e 0+e],c2);patch([0 0 1 1-e 0+e 0+e],[0 1 1 1-e 1-e 0+e],c3);plot([0 1 1 0 0],[0 0 1 1 0]);disp('weights');
  "IW{5,4}(6,:)'" : Constant  Value=[-0.9194845114805960673010076789068989455699920654296875;0.6809803679324393232974443890270777046680450439453125;-0.0505445538249365000638135825283825397491455078125;-0.463096400645814032515090730157680809497833251953125;-0.26512921079416162939423884381540119647979736328125;-0.3109052006854062799590110444114543497562408447265625;0.5037669258834684971049000523635186254978179931640625;-0.121970177314858485573267898871563374996185302734375;-0.584233207377109931002223675022833049297332763671875;-0.6908543554401764819061781963682733476161956787109375]
      mask Display: e = 0.06;c1 = [120 150 230]/255;c2 = ([120 150 230]+0)/383;c3 = ([120 150 230]+128)/383;patch([0 1 1 0],[0 0 1 1],c1);patch([0 1 1 1-e 1-e 0+e],[0 0 1 1-e 0+e 0+e],c2);patch([0 0 1 1-e 0+e 0+e],[0 1 1 1-e 1-e 0+e],c3);plot([0 1 1 0 0],[0 0 1 1 0]);disp('weights');
  "IW{5,4}(7,:)'" : Constant  Value=[-0.10033623539370876975862501012670691125094890594482421875;0.4053102734322273636990985323791392147541046142578125;-0.57394122859209828479976067683310247957706451416015625;0.59562123254917853643064518109895288944244384765625;-0.6960979286850286218424344042432494461536407470703125;-0.1439320984101896405693565839101211167871952056884765625;0.8185461096861441632199785090051591396331787109375;-0.1818066200584074199042561303940601646900177001953125;0.18866181353311706203612629906274378299713134765625;0.8631975272471363869186689043999649584293365478515625]
      mask Display: e = 0.06;c1 = [120 150 230]/255;c2 = ([120 150 230]+0)/383;c3 = ([120 150 230]+128)/383;patch([0 1 1 0],[0 0 1 1],c1);patch([0 1 1 1-e 1-e 0+e],[0 0 1 1-e 0+e 0+e],c2);patch([0 0 1 1-e 0+e 0+e],[0 1 1 1-e 1-e 0+e],c3);plot([0 1 1 0 0],[0 0 1 1 0]);disp('weights');
  "IW{5,4}(8,:)'" : Constant  Value=[0.3101619226920124816615498275496065616607666015625;0.0837156905538829765323072251703706569969654083251953125;-0.6504704523194277943076713199843652546405792236328125;0.2685122162222430830524899647571146488189697265625;-0.4544189259166360184138966360478661954402923583984375;-0.27360368085534736426467361525283195078372955322265625;0.2511362285026581542268786506610922515392303466796875;0.0396196768012935240932392844115383923053741455078125;0.3315910778638870848311626104987226426601409912109375;1.00416591011383804499246252817101776599884033203125]
      mask Display: e = 0.06;c1 = [120 150 230]/255;c2 = ([120 150 230]+0)/383;c3 = ([120 150 230]+128)/383;patch([0 1 1 0],[0 0 1 1],c1);patch([0 1 1 1-e 1-e 0+e],[0 0 1 1-e 0+e 0+e],c2);patch([0 0 1 1-e 0+e 0+e],[0 1 1 1-e 1-e 0+e],c3);plot([0 1 1 0 0],[0 0 1 1 0]);disp('weights');
  "IW{5,4}(9,:)'" : Constant  Value=[1.0243722660228569143470167546183802187442779541015625;0.9335708025525850661807680808124132454395294189453125;1.0711240327450524123520381181151606142520904541015625;0.778780788444122240576916738064028322696685791015625;0.52410706144383401028363778095808811485767364501953125;-0.74848790715246582561093191543477587401866912841796875;-0.1813830838923087274139334112987853586673736572265625;0.45664654471586185735532126273028552532196044921875;0.692070302564948836021585520938970148563385009765625;-0.6905352060005294223543614862137474119663238525390625]
      mask Display: e = 0.06;c1 = [120 150 230]/255;c2 = ([120 150 230]+0)/383;c3 = ([120 150 230]+128)/383;patch([0 1 1 0],[0 0 1 1],c1);patch([0 1 1 1-e 1-e 0+e],[0 0 1 1-e 0+e 0+e],c2);patch([0 0 1 1-e 0+e 0+e],[0 1 1 1-e 1-e 0+e],c3);plot([0 1 1 0 0],[0 0 1 1 0]);disp('weights');
  Mux : Mux  Inputs=10
      mask Display: e = 0.06;c1 = [120 150 230]/255;c2 = ([120 150 230]+0)/383;c3 = ([120 150 230]+128)/383;patch([0 1 1 0],[0 0 1 1],c1);patch([0 1 1 1-e 1-e 0+e],[0 0 1 1-e 0+e 0+e],c2);patch([0 0 1 1-e 0+e 0+e],[0 1 1 1-e 1-e 0+e],c3);plot([0 1 1 0 0],[0 0 1 1 0]);disp('Mux');
  dotprod{1..10} (10 alike) : neural/Weight Functions/dotprod
  "lz{5,4}" : Outport
      mask Display: e = 0.06;c1 = [120 230 180]/255;c2 = ([120 230 180]+0)/(256+128);c3 = ([120 230 180]+128)/(256+128);patch([0 1 1 0],[0 0 1 1],c1);patch([0 1 1 1-e 1-e 0+e],[0 0 1 1-e 0+e 0+e],c2);patch([0 0 1 1-e 0+e 0+e],[0 1 1 1-e 1-e 0+e],c3);plot([0 1 1 0 0],[0 0 1 1 0]);
  wires:
  "IW{5,4}(1,:)'"/1 -> dotprod1/1
  "ad{5,4}"/1 -> dotprod1/2, dotprod2/2, dotprod3/2, dotprod4/2, dotprod5/2, dotprod6/2, dotprod7/2, dotprod8/2, dotprod9/2, dotprod10/2
  dotprod1/1 -> Mux/1
  "IW{5,4}(2,:)'"/1 -> dotprod2/1
  dotprod2/1 -> Mux/2
  "IW{5,4}(3,:)'"/1 -> dotprod3/1
  dotprod3/1 -> Mux/3
  "IW{5,4}(4,:)'"/1 -> dotprod4/1
  dotprod4/1 -> Mux/4
  "IW{5,4}(5,:)'"/1 -> dotprod5/1
  dotprod5/1 -> Mux/5
  "IW{5,4}(6,:)'"/1 -> dotprod6/1
  dotprod6/1 -> Mux/6
  "IW{5,4}(7,:)'"/1 -> dotprod7/1
  dotprod7/1 -> Mux/7
  "IW{5,4}(8,:)'"/1 -> dotprod8/1
  dotprod8/1 -> Mux/8
  "IW{5,4}(9,:)'"/1 -> dotprod9/1
  dotprod9/1 -> Mux/9
  "IW{5,4}(10,:)'"/1 -> dotprod10/1
  dotprod10/1 -> Mux/10
  Mux/1 -> "lz{5,4}"/1

== system my_buck_nn_5_10/Feed-Forward Neural Network/Layer 6/Delays 1 ==
  "p{6}" : Inport  PortDimensions=10
      mask Display: e = 0.06;c1 = [120 230 180]/255;c2 = ([120 230 180]+0)/(256+128);c3 = ([120 230 180]+128)/(256+128);patch([0 1 1 0],[0 0 1 1],c1);patch([0 1 1 1-e 1-e 0+e],[0 0 1 1-e 0+e 0+e],c2);patch([0 0 1 1-e 0+e 0+e],[0 1 1 1-e 1-e 0+e],c3);plot([0 1 1 0 0],[0 0 1 1 0]);
  mux : Mux  Inputs=1
      mask Display: e = 0.06;c1 = [120 150 230]/255;c2 = ([120 150 230]+0)/383;c3 = ([120 150 230]+128)/383;patch([0 1 1 0],[0 0 1 1],c1);patch([0 1 1 1-e 1-e 0+e],[0 0 1 1-e 0+e 0+e],c2);patch([0 0 1 1-e 0+e 0+e],[0 1 1 1-e 1-e 0+e],c3);plot([0 1 1 0 0],[0 0 1 1 0]);disp('Mux')
  "pd{6,5}" : Outport
      mask Display: e = 0.06;c1 = [120 230 180]/255;c2 = ([120 230 180]+0)/(256+128);c3 = ([120 230 180]+128)/(256+128);patch([0 1 1 0],[0 0 1 1],c1);patch([0 1 1 1-e 1-e 0+e],[0 0 1 1-e 0+e 0+e],c2);patch([0 0 1 1-e 0+e 0+e],[0 1 1 1-e 1-e 0+e],c3);plot([0 1 1 0 0],[0 0 1 1 0]);
  wires:
  "p{6}"/1 -> mux/1
  mux/1 -> "pd{6,5}"/1

== system my_buck_nn_5_10/Feed-Forward Neural Network/Layer 6/LW{6,5} ==
  "ad{6,5}" : Inport  PortDimensions=10
      mask Display: e = 0.06;c1 = [120 230 180]/255;c2 = ([120 230 180]+0)/(256+128);c3 = ([120 230 180]+128)/(256+128);patch([0 1 1 0],[0 0 1 1],c1);patch([0 1 1 1-e 1-e 0+e],[0 0 1 1-e 0+e 0+e],c2);patch([0 0 1 1-e 0+e 0+e],[0 1 1 1-e 1-e 0+e],c3);plot([0 1 1 0 0],[0 0 1 1 0]);
  "IW{6,5}(1,:)'" : Constant  Value=[0.46823773230761978059177863542572595179080963134765625;-0.5934607550956148003251655609346926212310791015625;-1.1761911950469963183962818220607005059719085693359375;-0.95207485753430720620826832600869238376617431640625;-0.106319822873811364871698970091529190540313720703125;0.4983956159159770304967196352663449943065643310546875;-0.033933404132833543120906227841260260902345180511474609375;-0.701490757833318934189037463511340320110321044921875;1.179863702497538024971390768769197165966033935546875;-0.18543144713955239666347551974467933177947998046875]
      mask Display: e = 0.06;c1 = [120 150 230]/255;c2 = ([120 150 230]+0)/383;c3 = ([120 150 230]+128)/383;patch([0 1 1 0],[0 0 1 1],c1);patch([0 1 1 1-e 1-e 0+e],[0 0 1 1-e 0+e 0+e],c2);patch([0 0 1 1-e 0+e 0+e],[0 1 1 1-e 1-e 0+e],c3);plot([0 1 1 0 0],[0 0 1 1 0]);disp('weights');
  Mux : Mux  Inputs=1
      mask Display: e = 0.06;c1 = [120 150 230]/255;c2 = ([120 150 230]+0)/383;c3 = ([120 150 230]+128)/383;patch([0 1 1 0],[0 0 1 1],c1);patch([0 1 1 1-e 1-e 0+e],[0 0 1 1-e 0+e 0+e],c2);patch([0 0 1 1-e 0+e 0+e],[0 1 1 1-e 1-e 0+e],c3);plot([0 1 1 0 0],[0 0 1 1 0]);disp('Mux');
  dotprod1 : neural/Weight Functions/dotprod
  "lz{6,5}" : Outport
      mask Display: e = 0.06;c1 = [120 230 180]/255;c2 = ([120 230 180]+0)/(256+128);c3 = ([120 230 180]+128)/(256+128);patch([0 1 1 0],[0 0 1 1],c1);patch([0 1 1 1-e 1-e 0+e],[0 0 1 1-e 0+e 0+e],c2);patch([0 0 1 1-e 0+e 0+e],[0 1 1 1-e 1-e 0+e],c3);plot([0 1 1 0 0],[0 0 1 1 0]);
  wires:
  "IW{6,5}(1,:)'"/1 -> dotprod1/1
  "ad{6,5}"/1 -> dotprod1/2
  dotprod1/1 -> Mux/1
  Mux/1 -> "lz{6,5}"/1

== stateflow chart my_buck_nn_5_10/Buck Converter ==
  settings: updateMethod=CONTINUOUS
  state Discontinuous
    du:
    i_dot = 0;
    v_dot = a11o*v+b1o;
    t_dot = 1;
    i_out = i;
    v_out = v;
    mode_out=3;
  state Charging
    du:
    i_dot = a00c*i+a01c*v+b0c;
    v_dot = a10c*i+a11c*v+b1c;
    t_dot = 1;
    i_out = i;
    v_out = v;
    mode_out=2;
  state Discharging
    du:
    i_dot = a00o*i+a01o*v+b0o;
    v_dot = a10o*i+a11o*v+b1o;
    t_dot = 1;
    i_out = i;
    v_out = v;
    mode_out=1;
  Discharging -> Discontinuous [order 2] : [i < 0]
  Discontinuous -> Charging : [mode >= 1]
      | {t = 0;}
  Charging -> Discharging : [mode < 1]
  Discharging -> Charging [order 1] : [mode >= 1]
      | {t = 0;}
  (default) -> Charging : {i = i0;
      | v = v0;}
  data: t local double; i_out output double; v_out output double; i local double; a00o local double =a00o; a01o local double =a01o; a10o local double =a10o; a11o local double =a11o; a00c local double =a00c; a01c local double =a01c; a10c local double =a10c; a11c local double =a11c; b0o local double =b0o; b1o local double =b1o; b0c local double =b0c; b1c local double =b1c; v local double; i0 input double; v0 input double; mode input double =120; mode_out output double
  data t settings: updateMethod=SF_CONTINUOUS_TIME_DATA
  data i settings: updateMethod=SF_CONTINUOUS_TIME_DATA
  data v settings: updateMethod=SF_CONTINUOUS_TIME_DATA
